simulink model "fig_5_7"  (R2021b)
settings: Solver=ode23t  StartTime=0.0  StopTime=0.1  FixedStep=1e-5  RelTol=1e-4  EnableMultiTasking=on
undefined symbols (not defined in the file): Ts
libraries: spsSeriesRLCBranchLib x3, spsDiodeLib x1, spsMeanLib x1, spsMosfetLib x1, spsMultimeterLib x1, spsDCVoltageSourceLib x1, spspowerguiLib x1
settings Model: Creator=umi  LastModifiedBy=DELL
settings SolverCC: AlgebraicLoopSolver=TrustRegion
settings DataIOCC: LimitDataPoints=on  SaveFormat=Array  ReturnWorkspaceOutputs=off
settings OptimizationCC: LifeSpan=inf
settings DebuggingCC: SolverPrmCheckMsg=warning  SFUnexpectedBacktrackingDiag=warning  SFNoUnconditionalDefaultTransitionDiag=warning  SFExecutionAtInitializationDiag=none  SFMachineParentedDataDiag=warning  ArithmeticOperatorsInVariantConditions=warning
settings HardwareCC: ProdBitPerPointer=32  ProdBitPerSizeT=32  ProdBitPerPtrDiffT=32  ProdLargestAtomicFloat=None  ProdIntDivRoundTo=Undefined  ProdEndianess=Unspecified  ProdWordSize=32  ProdHWDeviceType=32-bit Generic
settings ModelReferenceCC: PropagateSignalLabelsOutOfModel=off
settings SFSimCC: SimUseLocalCustomCode=off  CustomCodeUndefinedFunction=UseInterfaceOnly
settings RTWCC: RTWUseLocalCustomCode=off
settings CodeAppCC: StateflowObjectComments=on
settings GRTTargetCC: TargetLangStandard=C89/C90 (ANSI)
settings ConfigComp: CovMetricSettings=dw  CovSaveCumulativeToWorkspaceVar=on  CovSaveSingleToWorkspaceVar=on  CovExternalEMLEnable=off  CovSFcnEnable=off
settings SimscapeCC: SimscapeNormalizeSystem=off

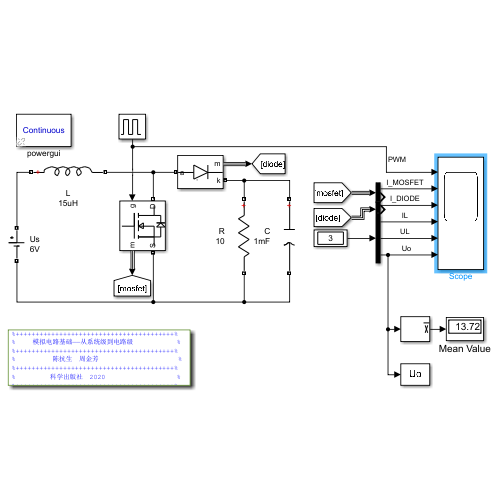
[thumbnail: Simulink's stored preview of the top-level diagram]
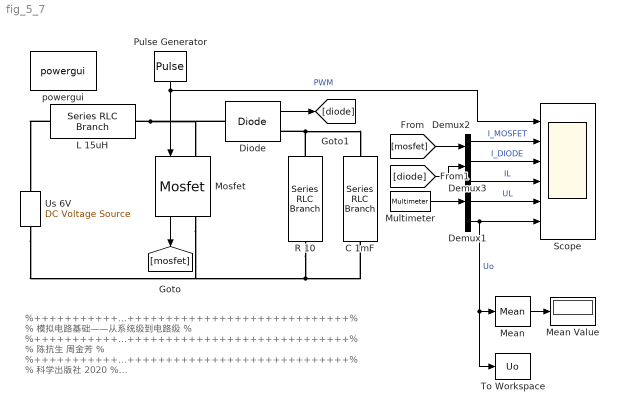
== system fig_5_7 ==
  note: %++++++++++++++++++++++++++++++++++++++++%
      | % 模拟电路基础——从系统级到电路级 %
      | %++++++++++++++++++++++++++++++++++++++++%
      | % 陈抗生 周金芳 %
      | %++++++++++++++++++++++++++++++++++++++++%
      | % 科学出版社 2020 %
      | %++++++++++++++++++++++++++++++++++++++++%
  C 1mF : spsSeriesRLCBranchLib/Series RLC Branch  LConnTagsString=__new0  RConnTagsString=__new0  BranchType=C  Resistance=1  Inductance=1e-3  SetiL0=off  InitialCurrent=0  Capacitance=1000e-6  Setx0=off  InitialVoltage=0  Measurements=Branch voltage
  Demux1 : Demux  Outputs=3
  Demux2 : Demux  Outputs=2
  Demux3 : Demux  Outputs=2
  Diode : spsDiodeLib/Diode  Ron=0.001  Lon=1e-8  Vf=0.7  IC=0  UseSnubber=off  Rs=1e5  Cs=Inf  Measurements=on
  L 15uH : spsSeriesRLCBranchLib/Series RLC Branch  LConnTagsString=__new0  RConnTagsString=__new0  BranchType=L  Resistance=1  Inductance=300e-6  SetiL0=off  InitialCurrent=0  Capacitance=1e-6  Setx0=off  InitialVoltage=0  Measurements=Branch voltage and current
  Mean : spsMeanLib/Mean  Freq=60  Vinit=0  Ts=0
  Mean Value : Display
      settings: Format=bank
  Mosfet : spsMosfetLib/Mosfet  Ron=0.1  Lon=0  Rd=0.01  Vfd=0  IC=0  Rs=1e5  Cs=inf  Measurements=on
  Multimeter : spsMultimeterLib/Multimeter  PhasorSimulation=off  OutputType=Complex  sel=[3 2 1]  L=4  Gain=[1 1 1]  yselected={'Ib: L 15uH','Ub: L 15uH','Ub: C 1mF'};  PSBOutputType=1  PSBequivalent=0  AxesSetting=[0,0.1,-100,100]  Display=0  SavedBlockNames=-11
  Pulse Generator : DiscretePulseGenerator  PulseType=Time based  Period=50e-5  PulseWidth=60
  R 10 : spsSeriesRLCBranchLib/Series RLC Branch  LConnTagsString=__new0  RConnTagsString=__new0  BranchType=R  Resistance=10  Inductance=1e-3  SetiL0=off  InitialCurrent=0  Capacitance=1e-6  Setx0=off  InitialVoltage=0  Measurements=Branch current
  Scope : Scope  NumInputPorts=6
  To Workspace : ToWorkspace  VariableName=Uo  SaveFormat=Timeseries  SampleTime=-1
  Us 6V : spsDCVoltageSourceLib/DC Voltage Source  Amplitude=6  Measurements=None
  powergui : spspowerguiLib/powergui  Priority=1  SimulationMode=Continuous  SampleTime=Ts  frequency=60  Iterations=50  frequencyindice=0  Pbase=100e6  ErrMax=1e-4  UnitsV=kV  UnitsW=MW  buscounter=0  FunctionMessages=off  echomessages=off  EnableUseOfTLC=off  CurrentSourceSwitches=off  DisableSnubberDevices=on  DisableRonSwitches=off  DisableVfSwitches=off  DisplayEquations=off  AutomaticDiscreteSolvers=off  SolverType=Tustin/Backward Euler (TBE)  Interpol=off  ExternalGateDelay=off  methode=off  Ts=100  x0status=blocks  SPID=on  SwTol=0  HookPort=off  NonlinearTolerance=1e-4  nMaxIteration=100  ContinueOnMaxIteration=off  RestoreLinks=warning  ResistiveCurrentMeasurement=off  Frange=[0:2:500]  Ylog=off  Xlog=on  ShowGrid=off  save=off  variable=ZData  structure=0  ZoomFFT=off  StartTime=0.0  cycles=1  DisplayStyle=1  fundamental=60  FreqAxis=off  MaxFrequency=1000  frequencyindicesteady=1  RmsSteady=1  display=off
  wires:
  Pulse Generator/1 -> Scope/1, Mosfet/1  "PWM"
  Mosfet/1 -> [mosfet]
  [mosfet] -> Demux2/1
  Demux2/1 -> Scope/2  "I_MOSFET"
  Diode/1 -> [diode]
  [diode] -> Demux3/1
  Demux3/1 -> Scope/3  "I_DIODE"
  Demux1/2 -> Scope/5  "UL"
  Multimeter/1 -> Demux1/1
  Demux1/1 -> Scope/4  "IL"
  Demux1/3 -> Mean/1, To Workspace/1, Scope/6  "Uo"
  Mean/1 -> Mean Value/1
  connections:
  L 15uH/RConn1 -- Diode/LConn1 -- Mosfet/LConn1
  R 10/RConn1 -- C 1mF/RConn1 -- Us 6V/LConn1 -- Mosfet/RConn1
  R 10/LConn1 -- C 1mF/LConn1 -- Diode/RConn1
  L 15uH/LConn1 -- Us 6V/RConn1
